simulink model "Dtm2020AtmosphereHarness"  (R2025a)
settings: Solver=ode45  StartTime=0  StopTime=200  RelTol=1e-09  AbsTol=1e-10
settings Model: Creator=juliankazmierski  LastModifiedBy=juliankazmierski

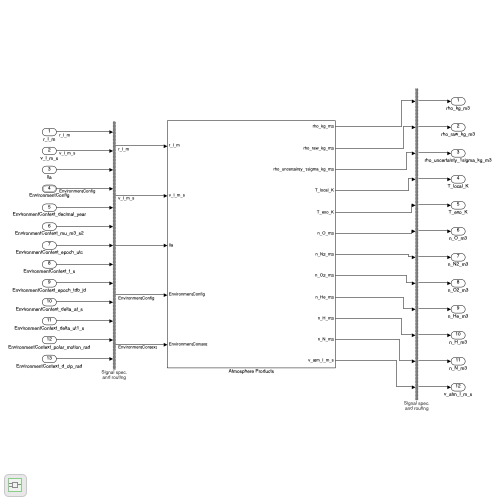
[thumbnail: Simulink's stored preview of the top-level diagram]
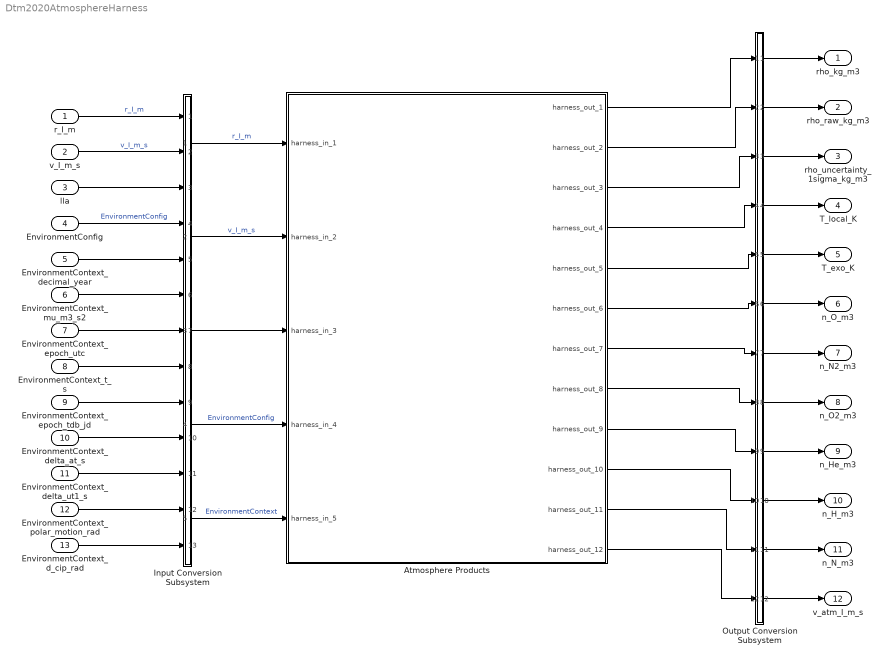
== system Dtm2020AtmosphereHarness ==
  r_I_m : Inport  OutDataTypeStr=double  PortDimensions=[3]  SampleTime=0
  v_I_m_s : Inport  Port=2  OutDataTypeStr=double  PortDimensions=[3]  SampleTime=0
  lla : Inport  Port=3  OutDataTypeStr=double  PortDimensions=[3]  SampleTime=0
  EnvironmentConfig : Inport  Port=4  OutDataTypeStr=Bus: EnvironmentConfigBus  PortDimensions=[1]  SampleTime=[-1, 0]  BusOutputAsStruct=on
  EnvironmentContext_decimal_year : Inport  Port=5  OutDataTypeStr=double  PortDimensions=[1]  SampleTime=0
  EnvironmentContext_mu_m3_s2 : Inport  Port=6  OutDataTypeStr=double  PortDimensions=[1, 1]  SampleTime=[-1, 0]
  EnvironmentContext_epoch_utc : Inport  Port=7  OutDataTypeStr=double  PortDimensions=[6, 1]  SampleTime=[-1, 0]
  EnvironmentContext_t_s : Inport  Port=8  OutDataTypeStr=double  PortDimensions=[1]  SampleTime=0
  EnvironmentContext_epoch_tdb_jd : Inport  Port=9  OutDataTypeStr=double  PortDimensions=[1, 1]  SampleTime=[-1, 0]
  EnvironmentContext_delta_at_s : Inport  Port=10  OutDataTypeStr=double  PortDimensions=[1]  SampleTime=[-1, 0]
  EnvironmentContext_delta_ut1_s : Inport  Port=11  OutDataTypeStr=double  PortDimensions=[1]  SampleTime=[-1, 0]
  EnvironmentContext_polar_motion_rad : Inport  Port=12  OutDataTypeStr=double  PortDimensions=[2]  SampleTime=[-1, 0]
  EnvironmentContext_d_cip_rad : Inport  Port=13  OutDataTypeStr=double  PortDimensions=[2]  SampleTime=[-1, 0]
  Atmosphere Products : Subsystem  Tag=__SL_testing_harness_stub_
  Input Conversion Subsystem : Subsystem  Tag=__SLT_ICS__  Description=|
      | Signal spec.
      | and routing
      settings: AttributesFormatString=%<Description>
  Output Conversion Subsystem : Subsystem  Tag=__SLT_OCS__  Description=|
      | Signal spec.
      | and routing
      settings: AttributesFormatString=%<Description>
  rho_kg_m3 : Outport
  rho_raw_kg_m3 : Outport  Port=2
  rho_uncertainty_1sigma_kg_m3 : Outport  Port=3
  T_local_K : Outport  Port=4
  T_exo_K : Outport  Port=5
  n_O_m3 : Outport  Port=6
  n_N2_m3 : Outport  Port=7
  n_O2_m3 : Outport  Port=8
  n_He_m3 : Outport  Port=9
  n_H_m3 : Outport  Port=10
  n_N_m3 : Outport  Port=11
  v_atm_I_m_s : Outport  Port=12
  wires:
  r_I_m/1 -> Input Conversion Subsystem/1(Inport_1)  "r_I_m"
  v_I_m_s/1 -> Input Conversion Subsystem/2(Inport_2)  "v_I_m_s"
  lla/1 -> Input Conversion Subsystem/3(Inport_3)
  EnvironmentConfig/1 -> Input Conversion Subsystem/4(Inport_4)  "EnvironmentConfig"
  EnvironmentContext_decimal_year/1 -> Input Conversion Subsystem/5(Inport_5)
  EnvironmentContext_mu_m3_s2/1 -> Input Conversion Subsystem/6(Inport_6)
  EnvironmentContext_epoch_utc/1 -> Input Conversion Subsystem/7(Inport_7)
  EnvironmentContext_t_s/1 -> Input Conversion Subsystem/8(Inport_8)
  EnvironmentContext_epoch_tdb_jd/1 -> Input Conversion Subsystem/9(Inport_9)
  EnvironmentContext_delta_at_s/1 -> Input Conversion Subsystem/10(Inport_10)
  EnvironmentContext_delta_ut1_s/1 -> Input Conversion Subsystem/11(Inport_11)
  EnvironmentContext_polar_motion_rad/1 -> Input Conversion Subsystem/12(Inport_12)
  EnvironmentContext_d_cip_rad/1 -> Input Conversion Subsystem/13(Inport_13)
  Output Conversion Subsystem/1(Outport_1) -> rho_kg_m3/1
  Output Conversion Subsystem/2(Outport_2) -> rho_raw_kg_m3/1
  Output Conversion Subsystem/3(Outport_3) -> rho_uncertainty_1sigma_kg_m3/1
  Output Conversion Subsystem/4(Outport_4) -> T_local_K/1
  Output Conversion Subsystem/5(Outport_5) -> T_exo_K/1
  Output Conversion Subsystem/6(Outport_6) -> n_O_m3/1
  Output Conversion Subsystem/7(Outport_7) -> n_N2_m3/1
  Output Conversion Subsystem/8(Outport_8) -> n_O2_m3/1
  Output Conversion Subsystem/9(Outport_9) -> n_He_m3/1
  Output Conversion Subsystem/10(Outport_10) -> n_H_m3/1
  Output Conversion Subsystem/11(Outport_11) -> n_N_m3/1
  Output Conversion Subsystem/12(Outport_12) -> v_atm_I_m_s/1
  Input Conversion Subsystem/1(Outport_1) -> Atmosphere Products/1(harness_in_1)  "r_I_m"
  Input Conversion Subsystem/2(Outport_2) -> Atmosphere Products/2(harness_in_2)  "v_I_m_s"
  Input Conversion Subsystem/3(Outport_3) -> Atmosphere Products/3(harness_in_3)
  Input Conversion Subsystem/4(Outport_4) -> Atmosphere Products/4(harness_in_4)  "EnvironmentConfig"
  Input Conversion Subsystem/5(Outport_5) -> Atmosphere Products/5(harness_in_5)  "EnvironmentContext"
  Atmosphere Products/1(harness_out_1) -> Output Conversion Subsystem/1(Inport_1)
  Atmosphere Products/2(harness_out_2) -> Output Conversion Subsystem/2(Inport_2)
  Atmosphere Products/3(harness_out_3) -> Output Conversion Subsystem/3(Inport_3)
  Atmosphere Products/4(harness_out_4) -> Output Conversion Subsystem/4(Inport_4)
  Atmosphere Products/5(harness_out_5) -> Output Conversion Subsystem/5(Inport_5)
  Atmosphere Products/6(harness_out_6) -> Output Conversion Subsystem/6(Inport_6)
  Atmosphere Products/7(harness_out_7) -> Output Conversion Subsystem/7(Inport_7)
  Atmosphere Products/8(harness_out_8) -> Output Conversion Subsystem/8(Inport_8)
  Atmosphere Products/9(harness_out_9) -> Output Conversion Subsystem/9(Inport_9)
  Atmosphere Products/10(harness_out_10) -> Output Conversion Subsystem/10(Inport_10)
  Atmosphere Products/11(harness_out_11) -> Output Conversion Subsystem/11(Inport_11)
  Atmosphere Products/12(harness_out_12) -> Output Conversion Subsystem/12(Inport_12)

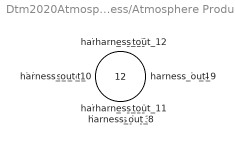
== system Dtm2020AtmosphereHarness/Atmosphere Products ==
  harness_in_1 : Inport
  harness_in_2 : Inport  Port=2
  harness_in_3 : Inport  Port=3
  harness_in_4 : Inport  Port=4
  harness_in_5 : Inport  Port=5
  harness_out_1 : Outport
  harness_out_2 : Outport  Port=2
  harness_out_3 : Outport  Port=3
  harness_out_4 : Outport  Port=4
  harness_out_5 : Outport  Port=5
  harness_out_6 : Outport  Port=6
  harness_out_7 : Outport  Port=7
  harness_out_8 : Outport  Port=8
  harness_out_9 : Outport  Port=9
  harness_out_10 : Outport  Port=10
  harness_out_11 : Outport  Port=11
  harness_out_12 : Outport  Port=12

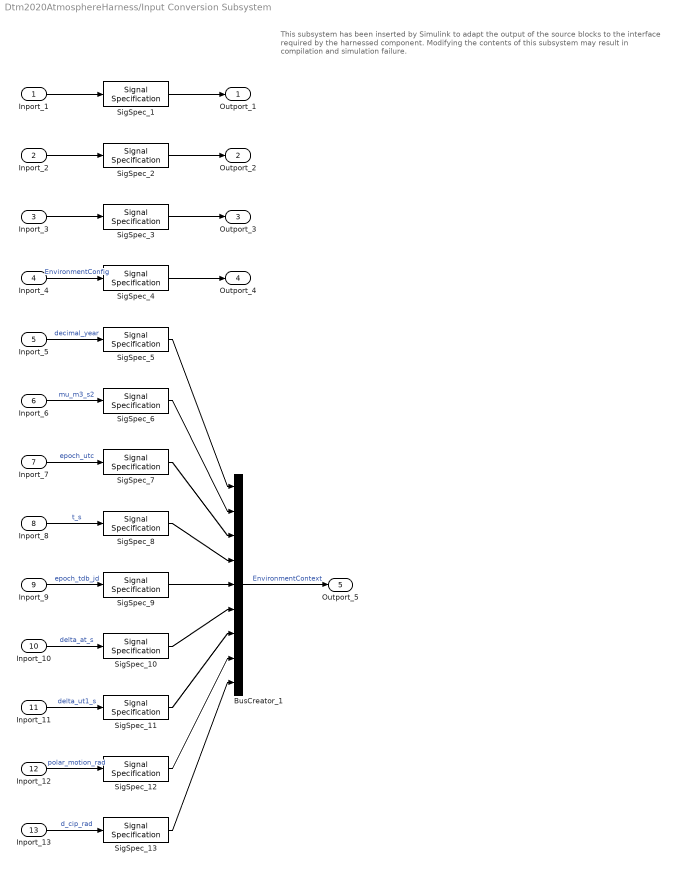
== system Dtm2020AtmosphereHarness/Input Conversion Subsystem ==
  note: This subsystem has been inserted by Simulink to adapt the output of the source blocks to the interface required by the harnessed component.
      |  Modifying the contents of this subsystem may result in compilation and simulation failure.
  Inport_1 : Inport
  Inport_2 : Inport  Port=2
  Inport_3 : Inport  Port=3
  Inport_4 : Inport  Port=4
  Inport_5 : Inport  Port=5
  Inport_6 : Inport  Port=6
  Inport_7 : Inport  Port=7
  Inport_8 : Inport  Port=8
  Inport_9 : Inport  Port=9
  Inport_10 : Inport  Port=10
  Inport_11 : Inport  Port=11
  Inport_12 : Inport  Port=12
  Inport_13 : Inport  Port=13
  BusCreator_1 : BusCreator  Inputs=9  OutDataTypeStr=Bus: EnvironmentContextBus
  SigSpec_1 : SignalSpecification  OutDataTypeStr=double  Unit=m  Dimensions=[3]  SampleTime=[0, 0]
  SigSpec_10 : SignalSpecification  OutDataTypeStr=double  Unit=sec  Dimensions=[1]  SampleTime=[-1, 0]
  SigSpec_11 : SignalSpecification  OutDataTypeStr=double  Unit=sec  Dimensions=[1]  SampleTime=[-1, 0]
  SigSpec_12 : SignalSpecification  OutDataTypeStr=double  Unit=rad  Dimensions=[2]  SampleTime=[-1, 0]
  SigSpec_13 : SignalSpecification  OutDataTypeStr=double  Unit=rad  Dimensions=[2]  SampleTime=[-1, 0]
  SigSpec_2 : SignalSpecification  OutDataTypeStr=double  Unit=m/s  Dimensions=[3]  SampleTime=[0, 0]
  SigSpec_3 : SignalSpecification  OutDataTypeStr=double  Dimensions=[3]  SampleTime=[0, 0]
  SigSpec_4 : SignalSpecification  OutDataTypeStr=Bus: EnvironmentConfigBus  Dimensions=[1]  SampleTime=[-1, 0]  BusOutputAsStruct=on
  SigSpec_5 : SignalSpecification  OutDataTypeStr=double  Unit=1  Dimensions=[1]  SampleTime=[0, 0]
  SigSpec_6 : SignalSpecification  OutDataTypeStr=double  Unit=m^3/s^2  Dimensions=[1, 1]  SampleTime=[-1, 0]
  SigSpec_7 : SignalSpecification  OutDataTypeStr=double  Unit=1  Dimensions=[6, 1]  SampleTime=[-1, 0]
  SigSpec_8 : SignalSpecification  OutDataTypeStr=double  Unit=s  Dimensions=[1]  SampleTime=[0, 0]
  SigSpec_9 : SignalSpecification  OutDataTypeStr=double  Unit=1  Dimensions=[1, 1]  SampleTime=[-1, 0]
  Outport_1 : Outport
  Outport_2 : Outport  Port=2
  Outport_3 : Outport  Port=3
  Outport_4 : Outport  Port=4
  Outport_5 : Outport  Port=5
  wires:
  SigSpec_1/1 -> Outport_1/1
  Inport_1/1 -> SigSpec_1/1
  SigSpec_2/1 -> Outport_2/1
  Inport_2/1 -> SigSpec_2/1
  SigSpec_3/1 -> Outport_3/1
  Inport_3/1 -> SigSpec_3/1
  SigSpec_4/1 -> Outport_4/1
  Inport_4/1 -> SigSpec_4/1  "EnvironmentConfig"
  BusCreator_1/1 -> Outport_5/1  "EnvironmentContext"
  SigSpec_5/1 -> BusCreator_1/1
  Inport_5/1 -> SigSpec_5/1  "decimal_year"
  SigSpec_6/1 -> BusCreator_1/2
  Inport_6/1 -> SigSpec_6/1  "mu_m3_s2"
  SigSpec_7/1 -> BusCreator_1/3
  Inport_7/1 -> SigSpec_7/1  "epoch_utc"
  SigSpec_8/1 -> BusCreator_1/4
  Inport_8/1 -> SigSpec_8/1  "t_s"
  SigSpec_9/1 -> BusCreator_1/5
  Inport_9/1 -> SigSpec_9/1  "epoch_tdb_jd"
  SigSpec_10/1 -> BusCreator_1/6
  Inport_10/1 -> SigSpec_10/1  "delta_at_s"
  SigSpec_11/1 -> BusCreator_1/7
  Inport_11/1 -> SigSpec_11/1  "delta_ut1_s"
  SigSpec_12/1 -> BusCreator_1/8
  Inport_12/1 -> SigSpec_12/1  "polar_motion_rad"
  SigSpec_13/1 -> BusCreator_1/9
  Inport_13/1 -> SigSpec_13/1  "d_cip_rad"

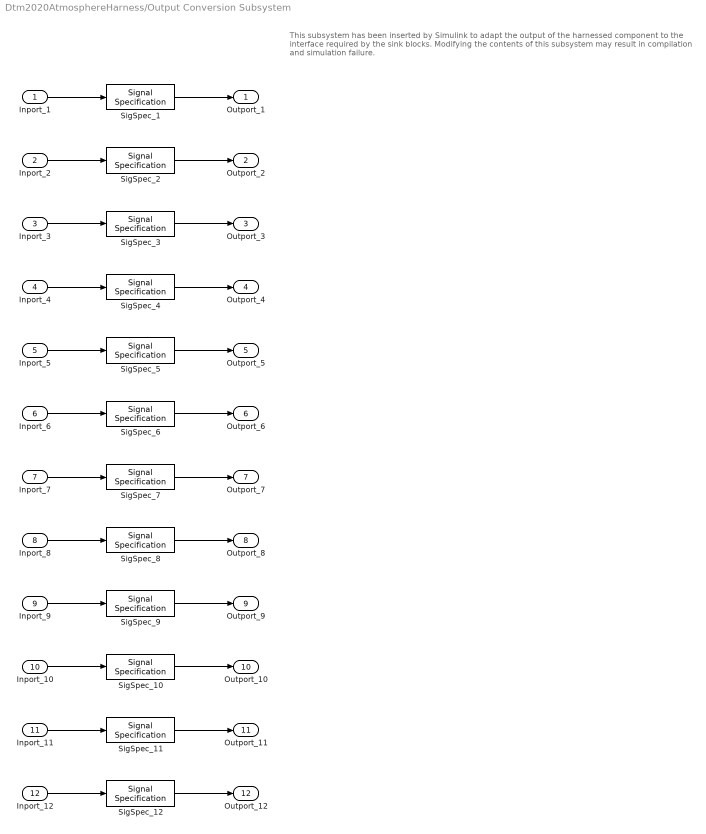
== system Dtm2020AtmosphereHarness/Output Conversion Subsystem ==
  note: This subsystem has been inserted by Simulink to adapt the output of the harnessed component to the interface required by the sink blocks.
      |  Modifying the contents of this subsystem may result in compilation and simulation failure.
  Inport_1 : Inport
  Inport_2 : Inport  Port=2
  Inport_3 : Inport  Port=3
  Inport_4 : Inport  Port=4
  Inport_5 : Inport  Port=5
  Inport_6 : Inport  Port=6
  Inport_7 : Inport  Port=7
  Inport_8 : Inport  Port=8
  Inport_9 : Inport  Port=9
  Inport_10 : Inport  Port=10
  Inport_11 : Inport  Port=11
  Inport_12 : Inport  Port=12
  SigSpec_1 : SignalSpecification  OutDataTypeStr=double  Unit=kg/m^3  Dimensions=[1]
  SigSpec_{6..11} (6 alike) : SignalSpecification  OutDataTypeStr=double  Unit=1/m^3  Dimensions=[1]
  SigSpec_12 : SignalSpecification  OutDataTypeStr=double  Unit=m/s  Dimensions=[3, 1]
  SigSpec_2 : SignalSpecification  OutDataTypeStr=double  Unit=kg/m^3  Dimensions=[1]
  SigSpec_3 : SignalSpecification  OutDataTypeStr=double  Unit=kg/m^3  Dimensions=[1]
  SigSpec_4 : SignalSpecification  OutDataTypeStr=double  Unit=K  Dimensions=[1]
  SigSpec_5 : SignalSpecification  OutDataTypeStr=double  Unit=K  Dimensions=[1]
  Outport_1 : Outport
  Outport_2 : Outport  Port=2
  Outport_3 : Outport  Port=3
  Outport_4 : Outport  Port=4
  Outport_5 : Outport  Port=5
  Outport_6 : Outport  Port=6
  Outport_7 : Outport  Port=7
  Outport_8 : Outport  Port=8
  Outport_9 : Outport  Port=9
  Outport_10 : Outport  Port=10
  Outport_11 : Outport  Port=11
  Outport_12 : Outport  Port=12
  wires:
  Inport_1/1 -> SigSpec_1/1
  SigSpec_1/1 -> Outport_1/1
  Inport_2/1 -> SigSpec_2/1
  SigSpec_2/1 -> Outport_2/1
  Inport_3/1 -> SigSpec_3/1
  SigSpec_3/1 -> Outport_3/1
  Inport_4/1 -> SigSpec_4/1
  SigSpec_4/1 -> Outport_4/1
  Inport_5/1 -> SigSpec_5/1
  SigSpec_5/1 -> Outport_5/1
  Inport_6/1 -> SigSpec_6/1
  SigSpec_6/1 -> Outport_6/1
  Inport_7/1 -> SigSpec_7/1
  SigSpec_7/1 -> Outport_7/1
  Inport_8/1 -> SigSpec_8/1
  SigSpec_8/1 -> Outport_8/1
  Inport_9/1 -> SigSpec_9/1
  SigSpec_9/1 -> Outport_9/1
  Inport_10/1 -> SigSpec_10/1
  SigSpec_10/1 -> Outport_10/1
  Inport_11/1 -> SigSpec_11/1
  SigSpec_11/1 -> Outport_11/1
  Inport_12/1 -> SigSpec_12/1
  SigSpec_12/1 -> Outport_12/1
